simulink model "sensorExpoler"  (R2026a)
settings: Solver=FixedStepDiscrete  StopTime=10  FixedStep=0.001
undefined symbols (not defined in the file or in its folder): Blocking, Non
libraries: amg_usbconverter_n_connect_lib x2
settings Model: Creator=pboon  LastModifiedBy=raksa

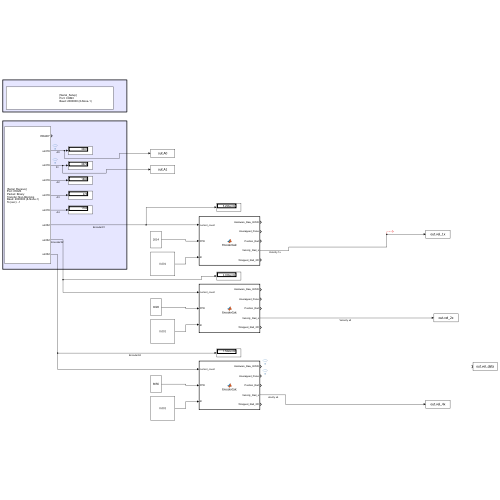
[thumbnail: Simulink's stored preview of the top-level diagram]
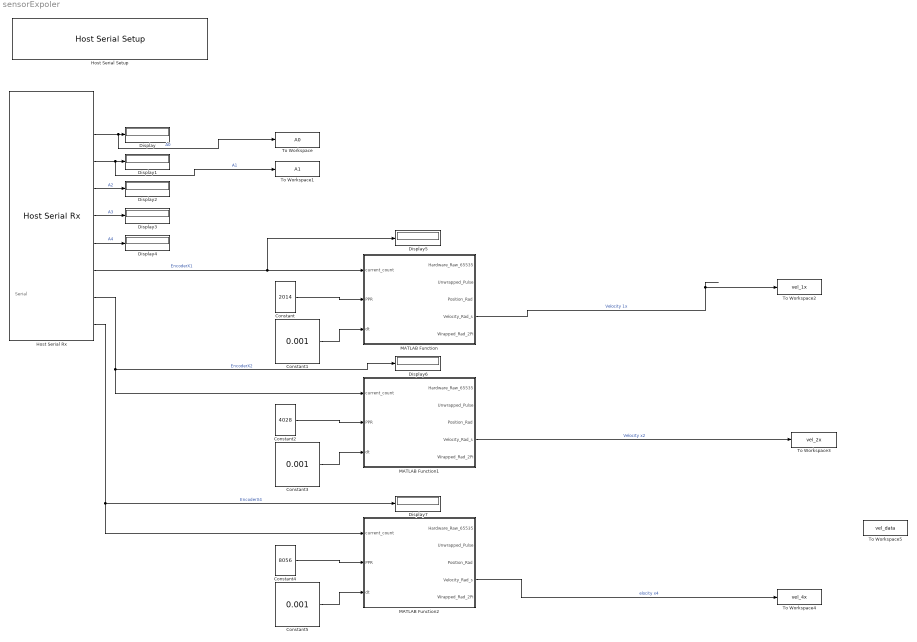
== system sensorExpoler ==
  note: Serial
  Constant : Constant  Value=2014
  Constant1 : Constant  Value=0.001
  Constant2 : Constant  Value=4028
  Constant3 : Constant  Value=0.001
  Constant4 : Constant  Value=8056
  Constant5 : Constant  Value=0.001
  Display{,1..7} (8 alike) : Display
  Host Serial Rx : amg_usbconverter_n_connect_lib/Host Serial Rx  conf=rx  port=<auto>  baudrate=2000000  databits=8  parity=None  stopbit=1  flowcontrol=None  transfer=Non-Blocking  timeout=5  packetmode=Binary  enableinitialvalues=off  initialvalues=[]  binheader='25'  binterminator='4E 4E'  porttype_double=0  porttype_single=0  porttype_int8=0  porttype_uint8=0  porttype_int16=0  porttype_uint16=5  porttype_int32=0  porttype_uint32=3  asciiformat='%d,%f'  rx_asciiterminator="CRLF (0x0D 0x0A - \"\\r\\n\")"  tx_asciiterminator="CRLF (0x0D 0x0A - \"\\r\\n\")"  sampletime=0.001  enablecustomportlabel=off  cinputportlabel=0  coutputportlabel=A  portpinstr=0  blockid=HostSerialRx  inputporttype=[]  inputportwidth=[]  inputportlabel={}  outputporttype=[3 5 5 5 5 5 7 7 7]  outputportwidth=[1 1 1 1 1 1 1 1 1]  outputportlabel={'READY','uint16','uint16','uint16','uint16','uint16','uint32','uint32','uint32'}  compat=0  optionstring=[]  autoport='COM3'
  Host Serial Setup : amg_usbconverter_n_connect_lib/Host Serial Setup  conf=setup  port=<auto>  baudrate=2000000  databits=8  parity=None  stopbit=1  flowcontrol=None  transfer=Blocking  timeout=2  packetmode=Binary  initialvalues=[]  binheader='7E 7E'  binterminator='03 03'  porttype_double=0  porttype_single=1  porttype_int8=0  porttype_uint8=0  porttype_int16=0  porttype_uint16=0  porttype_int32=0  porttype_uint32=2  asciiformat='%d %u %x'  rx_asciiterminator="CRLF (0x0D 0x0A - \"\\r\\n\")"  tx_asciiterminator="CRLF (0x0D 0x0A - \"\\r\\n\")"  sampletime=-1  enablecustomportlabel=off  cinputportlabel=0  coutputportlabel=A  portpinstr=0  blockid=HostSerialSetup  inputporttype=[]  inputportwidth=[]  inputportlabel={}  outputporttype=[]  outputportwidth=[]  outputportlabel={}  compat=0  optionstring=[]  autoport='COM3'
  MATLAB Function : MATLAB Function  TreatAsAtomicUnit=on
  MATLAB Function1 : MATLAB Function  TreatAsAtomicUnit=on
  MATLAB Function2 : MATLAB Function  TreatAsAtomicUnit=on
  To Workspace : ToWorkspace  VariableName=A0  SaveFormat=Timeseries  SampleTime=-1
  To Workspace1 : ToWorkspace  VariableName=A1  SaveFormat=Timeseries  SampleTime=-1
  To Workspace2 : ToWorkspace  VariableName=vel_1x  SaveFormat=Timeseries  SampleTime=-1
  To Workspace3 : ToWorkspace  VariableName=vel_2x  SaveFormat=Timeseries  SampleTime=-1
  To Workspace4 : ToWorkspace  VariableName=vel_4x  SaveFormat=Timeseries  SampleTime=-1
  To Workspace5 : ToWorkspace  VariableName=vel_data  SaveFormat=Timeseries  SampleTime=-1
  wires:
  Host Serial Rx/2 -> To Workspace/1, Display/1  "A0"
  Host Serial Rx/3 -> To Workspace1/1, Display1/1  "A1"
  Host Serial Rx/4 -> Display2/1  "A2"
  Host Serial Rx/5 -> Display3/1  "A3"
  Host Serial Rx/6 -> Display4/1  "A4"
  Host Serial Rx/7 -> Display5/1, MATLAB Function/1(current_count)  "EncoderX1"
  Host Serial Rx/8 -> MATLAB Function1/1(current_count), Display6/1  "EncoderX2"
  Host Serial Rx/9 -> MATLAB Function2/1(current_count), Display7/1  "EncoderX4"
  Constant1/1 -> MATLAB Function/3(dt)
  Constant/1 -> MATLAB Function/2(PPR)
  Constant2/1 -> MATLAB Function1/2(PPR)
  Constant3/1 -> MATLAB Function1/3(dt)
  Constant4/1 -> MATLAB Function2/2(PPR)
  Constant5/1 -> MATLAB Function2/3(dt)
  MATLAB Function/4(Velocity_Rad_s) -> To Workspace2/1  "Velocity 1x"
  MATLAB Function1/4(Velocity_Rad_s) -> To Workspace3/1  "Velocity x2"
  MATLAB Function2/4(Velocity_Rad_s) -> To Workspace4/1  "elocity x4"

== matlab function sensorExpoler/MATLAB Function1 ==
  data: Hardware_Raw_65535 output; Unwrapped_Pulse output; current_count input; Position_Rad output; PPR input; dt input; Velocity_Rad_s output; Wrapped_Rad_2Pi output
function [Hardware_Raw_65535, Unwrapped_Pulse, Position_Rad, Velocity_Rad_s, Wrapped_Rad_2Pi] = EncoderCalc(current_count, PPR, dt)
    persistent prev_count
    persistent n_pulse 
    persistent prev_n_pulse 
    persistent startup_ticks
    persistent prev_vel 
    
    if isempty(prev_count)
        prev_count = current_count;
        n_pulse = 0;
        prev_n_pulse = 0;
        startup_ticks = 0;
        prev_vel = 0; 
    end
    
    startup_ticks = startup_ticks + 1;
    
    % 1. Auto-Homing
    if startup_ticks < 100
        n_pulse = 0;            
        prev_n_pulse = 0;       
        prev_count = current_count; 
        prev_vel = 0;
    end
    
    % 2. อ่านค่าดิบ
    Hardware_Raw_65535 = mod(current_count, 65536);
    
    % 3. Unwrapping (แก้ Overflow)
    delta_count = double(current_count) - double(prev_count);
    
    if delta_count < -32768
        delta_count = delta_count + 65536; 
    elseif delta_count > 32768
        delta_count = delta_count - 65536; 
    end
    
    n_pulse = n_pulse + delta_count; 
    Unwrapped_Pulse = n_pulse;
    
    % 4. คำนวณ Position
    res_theta_rad = (2 * pi) / double(PPR);
    Position_Rad = res_theta_rad * n_pulse; 
    
    % 5. คำนวณ Velocity 
    d_dt_n_pulse = (n_pulse - prev_n_pulse) / double(dt); 
    raw_vel = res_theta_rad * d_dt_n_pulse; 
    
    % ==========================================
    % 🌟 SMART SPIKE REJECTION (ดักจากความเร่ง) 🌟
    % ==========================================
    % ขีดจำกัด: ห้ามความเร็วเปลี่ยนแปลงเกิน 10 rad/s ภายใน 0.001 วินาที
    max_delta_vel = 10;
    
    if abs(raw_vel - prev_vel) > max_delta_vel 
        % ถ้ากระชากแรงผิดมนุษย์ (USB สะดุด) -> ให้ใช้ค่าความเร็วเดิมไปก่อน
        Velocity_Rad_s = prev_vel; 
    else
        % ถ้าขยับตามจังหวะปกติของมนุษย์ -> รับค่าความเร็วใหม่มาใช้
        Velocity_Rad_s = raw_vel;  
    end
    
    % อัปเดตเก็บความเร็วปัจจุบันไว้เทียบลูปถัดไป
    prev_vel = Velocity_Rad_s;        
    % ==========================================
    
    Wrapped_Rad_2Pi = mod(Position_Rad, 2*pi);
    
    % อัปเดตตัวแปรระบบ
    prev_count = current_count;
    prev_n_pulse = n_pulse;
end

== matlab function sensorExpoler/MATLAB Function ==
  data: Hardware_Raw_65535 output; Unwrapped_Pulse output; current_count input; Position_Rad output; PPR input; dt input; Velocity_Rad_s output; Wrapped_Rad_2Pi output
function [Hardware_Raw_65535, Unwrapped_Pulse, Position_Rad, Velocity_Rad_s, Wrapped_Rad_2Pi] = EncoderCalc(current_count, PPR, dt)
    persistent prev_count
    persistent n_pulse 
    persistent prev_n_pulse 
    persistent startup_ticks
    persistent prev_vel 
    
    if isempty(prev_count)
        prev_count = current_count;
        n_pulse = 0;
        prev_n_pulse = 0;
        startup_ticks = 0;
        prev_vel = 0; 
    end
    
    startup_ticks = startup_ticks + 1;
    
    % 1. Auto-Homing
    if startup_ticks < 100
        n_pulse = 0;            
        prev_n_pulse = 0;       
        prev_count = current_count; 
        prev_vel = 0;
    end
    
    % 2. อ่านค่าดิบ
    Hardware_Raw_65535 = mod(current_count, 65536);
    
    % 3. Unwrapping (แก้ Overflow)
    delta_count = double(current_count) - double(prev_count);
    
    if delta_count < -32768
        delta_count = delta_count + 65536; 
    elseif delta_count > 32768
        delta_count = delta_count - 65536; 
    end
    
    n_pulse = n_pulse + delta_count; 
    Unwrapped_Pulse = n_pulse;
    
    % 4. คำนวณ Position
    res_theta_rad = (2 * pi) / double(PPR);
    Position_Rad = res_theta_rad * n_pulse; 
    
    % 5. คำนวณ Velocity 
    d_dt_n_pulse = (n_pulse - prev_n_pulse) / double(dt); 
    raw_vel = res_theta_rad * d_dt_n_pulse; 
    
    % ==========================================
    % 🌟 SMART SPIKE REJECTION (ดักจากความเร่ง) 🌟
    % ==========================================
    % ขีดจำกัด: ห้ามความเร็วเปลี่ยนแปลงเกิน 10 rad/s ภายใน 0.001 วินาที
    max_delta_vel = 10;
    
    if abs(raw_vel - prev_vel) > max_delta_vel 
        % ถ้ากระชากแรงผิดมนุษย์ (USB สะดุด) -> ให้ใช้ค่าความเร็วเดิมไปก่อน
        Velocity_Rad_s = prev_vel; 
    else
        % ถ้าขยับตามจังหวะปกติของมนุษย์ -> รับค่าความเร็วใหม่มาใช้
        Velocity_Rad_s = raw_vel;  
    end
    
    % อัปเดตเก็บความเร็วปัจจุบันไว้เทียบลูปถัดไป
    prev_vel = Velocity_Rad_s;        
    % ==========================================
    
    Wrapped_Rad_2Pi = mod(Position_Rad, 2*pi);
    
    % อัปเดตตัวแปรระบบ
    prev_count = current_count;
    prev_n_pulse = n_pulse;
end

== matlab function sensorExpoler/MATLAB Function2 ==
  data: Hardware_Raw_65535 output; Unwrapped_Pulse output; current_count input; Position_Rad output; PPR input; dt input; Velocity_Rad_s output; Wrapped_Rad_2Pi output
function [Hardware_Raw_65535, Unwrapped_Pulse, Position_Rad, Velocity_Rad_s, Wrapped_Rad_2Pi] = EncoderCalc(current_count, PPR, dt)
    persistent prev_count
    persistent n_pulse 
    persistent prev_n_pulse 
    persistent startup_ticks
    persistent prev_vel 
    
    if isempty(prev_count)
        prev_count = current_count;
        n_pulse = 0;
        prev_n_pulse = 0;
        startup_ticks = 0;
        prev_vel = 0; 
    end
    
    startup_ticks = startup_ticks + 1;
    
    % 1. Auto-Homing
    if startup_ticks < 100
        n_pulse = 0;            
        prev_n_pulse = 0;       
        prev_count = current_count; 
        prev_vel = 0;
    end
    
    % 2. อ่านค่าดิบ
    Hardware_Raw_65535 = mod(current_count, 65536);
    
    % 3. Unwrapping (แก้ Overflow)
    delta_count = double(current_count) - double(prev_count);
    
    if delta_count < -32768
        delta_count = delta_count + 65536; 
    elseif delta_count > 32768
        delta_count = delta_count - 65536; 
    end
    
    n_pulse = n_pulse + delta_count; 
    Unwrapped_Pulse = n_pulse;
    
    % 4. คำนวณ Position
    res_theta_rad = (2 * pi) / double(PPR);
    Position_Rad = res_theta_rad * n_pulse; 
    
    % 5. คำนวณ Velocity 
    d_dt_n_pulse = (n_pulse - prev_n_pulse) / double(dt); 
    raw_vel = res_theta_rad * d_dt_n_pulse; 
    
    % ==========================================
    % 🌟 SMART SPIKE REJECTION (ดักจากความเร่ง) 🌟
    % ==========================================
    % ขีดจำกัด: ห้ามความเร็วเปลี่ยนแปลงเกิน 10 rad/s ภายใน 0.001 วินาที
    max_delta_vel = 10;
    
    if abs(raw_vel - prev_vel) > max_delta_vel 
        % ถ้ากระชากแรงผิดมนุษย์ (USB สะดุด) -> ให้ใช้ค่าความเร็วเดิมไปก่อน
        Velocity_Rad_s = prev_vel; 
    else
        % ถ้าขยับตามจังหวะปกติของมนุษย์ -> รับค่าความเร็วใหม่มาใช้
        Velocity_Rad_s = raw_vel;  
    end
    
    % อัปเดตเก็บความเร็วปัจจุบันไว้เทียบลูปถัดไป
    prev_vel = Velocity_Rad_s;        
    % ==========================================
    
    Wrapped_Rad_2Pi = mod(Position_Rad, 2*pi);
    
    % อัปเดตตัวแปรระบบ
    prev_count = current_count;
    prev_n_pulse = n_pulse;
end
